simulink model "mavsim_chap4"  (R2018b)
settings: Solver=ode45  StartTime=0.0  StopTime=10000  RelTol=1e-3  EnableMultiTasking=on
PreLoadFcn:
  | param
  | aerosonde
InitFcn:
  | param
  | aerosonde
values from neighbouring files (symbols this model uses):
  q = uu(11)    [drawVehicle.m]    (also in forces_moments.m = x(11))
  r = uu(12)    [drawVehicle.m]    (also in forces_moments.m = x(12))
undefined symbols (not defined in the file or in its folder): drawVehicle, forces_moments, HDBK, Light, MIL, Newton, P, plotmavstatevariables, Raphson, sigbuilder_block
libraries: simulink x4, aerolibwind2 x2, aerolibobsolete x1
settings Model: Creator=beard  LastModifiedBy=xinyizhao
settings DataIOCC: LimitDataPoints=on  SaveFormat=Array  SignalLoggingSaveFormat=ModelDataLogs
settings OptimizationCC: ExpressionDepthLimit=2147483647  InitFltsAndDblsToZero=on  LifeSpan=inf
settings DebuggingCC: UnderspecifiedInitializationDetection=Classic  MergeDetectMultiDrivingBlocksExec=none  SolverPrmCheckMsg=warning  FcnCallInpInsideContextMsg=warning  StateNameClashWarn=warning  LibraryContextMissingDiagnostic=none  SFUnexpectedBacktrackingDiag=warning  SFNoUnconditionalDefaultTransitionDiag=warning  SFExecutionAtInitializationDiag=none
settings HardwareCC: ProdBitPerPointer=32  ProdBitPerSizeT=32  ProdBitPerPtrDiffT=32  ProdLargestAtomicFloat=None  ProdIntDivRoundTo=Undefined  ProdEndianess=Unspecified  ProdWordSize=32  ProdHWDeviceType=32-bit Generic
settings ModelReferenceCC: PropagateSignalLabelsOutOfModel=off
settings SFSimCC: SimUseLocalCustomCode=off
settings RTWCC: RTWUseLocalCustomCode=off
settings CodeAppCC: StateflowObjectComments=on
settings GRTTargetCC: TargetLangStandard=C89/C90 (ANSI)  GeneratePreprocessorConditionals=Disable all  CombineOutputUpdateFcns=off  GRTInterface=on
settings ConfigComp: CovMetricSettings=dw  CovHtmlReporting=on  CovSaveCumulativeToWorkspaceVar=on  CovSaveSingleToWorkspaceVar=on  CovExternalEMLEnable=off  CovSFcnEnable=off

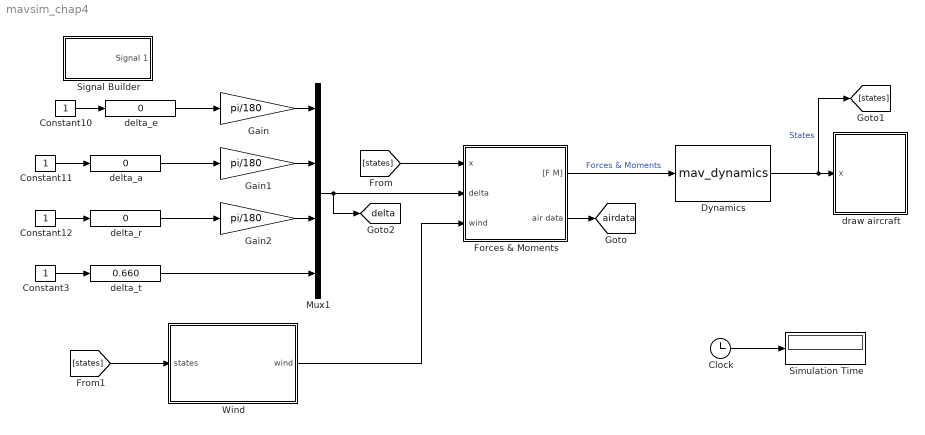
== system mavsim_chap4 ==
  Clock : Clock
  Constant{3,10..12} (4 alike) : Constant
  Dynamics : S-Function  FunctionName=mav_dynamics  Parameters=P  SFunctionDeploymentMode=off  EnableBusSupport=off
  Forces & Moments : Subsystem
  Gain : Gain  Gain=pi/180
  Gain1 : Gain  Gain=pi/180
  Gain2 : Gain  Gain=pi/180
  Mux1 : Mux
  Signal Builder : Subsystem  Tag=STV Subsys  LoadFcn=sigbuilder_block('load');  StartFcn=sigbuilder_block('start');  StopFcn=sigbuilder_block('stop');  ClipboardFcn=sigbuilder_block('clipboard');  mask(Sigbuilder block){tuvar=[0:10]}
      mask help: Simulink:masks:SigbuilderBlock_MD
      mask init:
      | if ~strcmp(get_param(bdroot(gcbh),'SimulationStatus'),'stopped') tuvar = sigbuilder_block('maskInit'); end
      settings: CopyFcn=sigbuilder_block('copy');  DeleteFcn=sigbuilder_block('delete');  ModelCloseFcn=sigbuilder_block('modelClose');  PreSaveFcn=sigbuilder_block('preSave');  PauseFcn=sigbuilder_block('pause');  ContinueFcn=sigbuilder_block('continue');  NameChangeFcn=sigbuilder_block('namechange');  OpenFcn=sigbuilder_block('open',[382.5 81 550.5 358.5 ]);  CloseFcn=sigbuilder_block('close');
      mask Display: plot(0, 0, 100, 100,[2, 2, 32, 32, 2], [68, 8, 8, 68, 68],[32, 2], [38, 38], [32, 19, 2],[53, 60, 44], [32, 17, 17, 2],[16, 16, 31, 31]);txt = getActiveGroup(gcbh);text(2, 100, txt,'verticalAlignment', 'top');
  Simulation Time : Display
  Wind : Subsystem
  delta_a : simulink/Math Operations/Slider Gain  gain=0  low=-45  high=45
  delta_e : simulink/Math Operations/Slider Gain  gain=0  low=-45  high=45
  delta_r : simulink/Math Operations/Slider Gain  gain=0  low=-45  high=45
  delta_t : simulink/Math Operations/Slider Gain  gain=0.660  low=0  high=1
  draw aircraft : Subsystem
      mask Display: image(imread('tv.jpg'))
  tag scope: airdata=global, delta=global
  wires:
  Constant10/1 -> delta_e/1
  Constant11/1 -> delta_a/1
  Constant12/1 -> delta_r/1
  Dynamics/1 -> [states], draw aircraft/1(x)  "States"
  Constant3/1 -> delta_t/1
  delta_t/1 -> Mux1/4
  Mux1/1 -> [delta], Forces & Moments/2(delta)
  Forces & Moments/1("[F M]") -> Dynamics/1  "Forces & Moments"
  Clock/1 -> Simulation Time/1
  Wind/1(wind) -> Forces & Moments/3(wind)
  Forces & Moments/2(air data) -> [airdata]
  Gain/1 -> Mux1/1
  Gain1/1 -> Mux1/2
  Gain2/1 -> Mux1/3
  [states] -> Forces & Moments/1(x)
  [states] -> Wind/1(states)
  delta_e/1 -> Gain/1
  delta_a/1 -> Gain1/1
  delta_r/1 -> Gain2/1

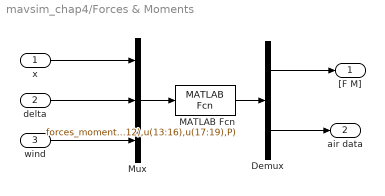
== system mavsim_chap4/Forces & Moments ==
  x : Inport
  delta : Inport  Port=2
  wind : Inport  Port=3
  Demux : Demux  Outputs=[6;6]
  MATLAB Fcn : MATLABFcn  MATLABFcn=forces_moments(u(1:12),u(13:16),u(17:19),P)  OutputDimensions=12
  Mux : Mux  Inputs=3
  "[F M]" : Outport
  air data : Outport  Port=2
  wires:
  x/1 -> Mux/1
  delta/1 -> Mux/2
  wind/1 -> Mux/3
  MATLAB Fcn/1 -> Demux/1
  Demux/1 -> "[F M]"/1
  Mux/1 -> MATLAB Fcn/1
  Demux/2 -> air data/1

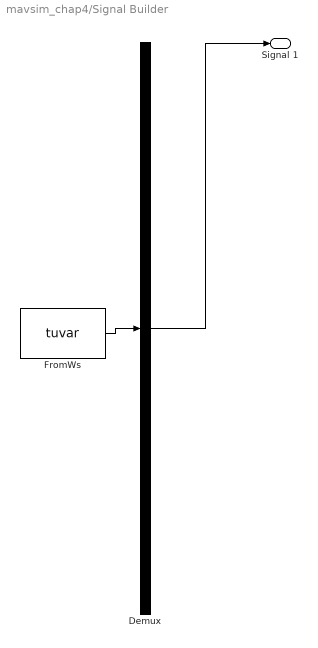
== system mavsim_chap4/Signal Builder ==
  Demux : Demux  Tag=STV Demux  Outputs=1
  FromWs : FromWorkspace  Tag=STV FromWs  VariableName=tuvar  SampleTime=0
      SigBuilderData=|
      | common.afterFinalStr = 'Extrapolate'
      | common.sampleTime = 0
      | dataSet.timeRange = [0 20]
      | dataSet.name = 'Group 1'
      | sbobj.Groups.Name = 'Group 1'
      | sbobj.Groups.Signals.Name = 'Signal 1'
      | sbobj.Groups.Signals.XData = [0 10 10 15 15 20]
      | sbobj.Groups.Signals.YData = [0 0 5 5 0 0]
      | sbobj.Groups.TimeRange = [0 20]
  Signal 1 : Outport  Tag=STV Outport
  wires:
  Demux/1 -> Signal 1/1
  FromWs/1 -> Demux/1

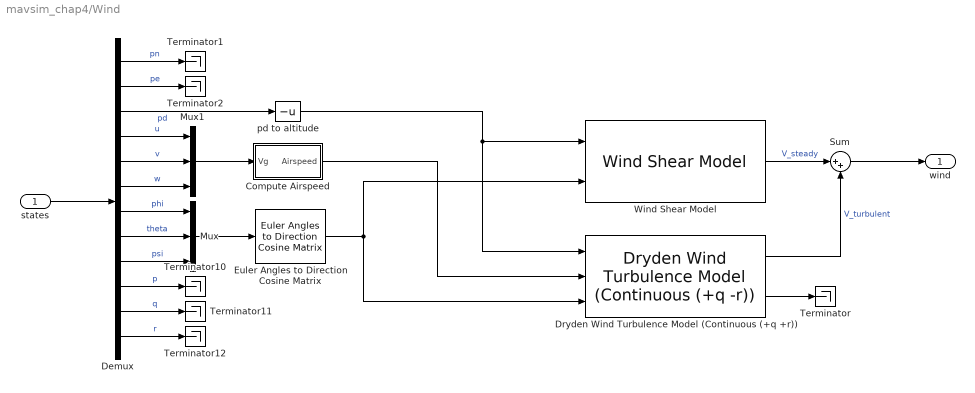
== system mavsim_chap4/Wind ==
  states : Inport
  Compute Airspeed : Subsystem
  Demux : Demux  Outputs=12
  Dryden Wind Turbulence Model (Continuous (+q +r)) : aerolibwind2/Dryden Wind Turbulence Model  (Continuous (+q -r))  units=Metric (MKS)  spec=MIL-HDBK-1797  model=Continuous Dryden (+q +r)  W20=P.w_mag  Wdeg=P.w_dir  TurbProb=10^-2 - Light  L_high=533.4  Wingspan=P.b  ts=0.1  Seed=[23341 23342 0 23344]  T_on=off
      settings: SourceProductName=Aerospace Blockset
  Euler Angles to Direction Cosine Matrix : aerolibobsolete/Euler Angles to  Direction Cosine Matrix
      settings: SourceProductName=Aerospace Blockset  SourceProductBaseCode=AE
  Mux : Mux  Inputs=3
  Mux1 : Mux  Inputs=3
  Sum : Sum  Inputs=|++
  Terminator{,1..2,10..12} (6 alike) : Terminator
  Wind Shear Model : aerolibwind2/Wind Shear Model  units=Metric (MKS)  phase=Category C - Terminal Flight Phase  W_20=P.w_mag  Wdeg=P.w_dir
      settings: SourceProductName=Aerospace Blockset
  pd to altitude : UnaryMinus
  wind : Outport
  wires:
  Dryden Wind Turbulence Model (Continuous (+q +r))/2 -> Terminator/1
  Euler Angles to Direction Cosine Matrix/1 -> Dryden Wind Turbulence Model (Continuous (+q +r))/3, Wind Shear Model/2
  Wind Shear Model/1 -> Sum/1  "V_steady"
  Compute Airspeed/1(Airspeed) -> Dryden Wind Turbulence Model (Continuous (+q +r))/2
  pd to altitude/1 -> Wind Shear Model/1, Dryden Wind Turbulence Model (Continuous (+q +r))/1
  Dryden Wind Turbulence Model (Continuous (+q +r))/1 -> Sum/2  "V_turbulent"
  states/1 -> Demux/1
  Demux/1 -> Terminator1/1  "pn"
  Demux/2 -> Terminator2/1  "pe"
  Demux/3 -> pd to altitude/1  "pd"
  Demux/4 -> Mux1/1  "u"
  Demux/5 -> Mux1/2  "v"
  Demux/6 -> Mux1/3  "w"
  Demux/7 -> Mux/1  "phi"
  Demux/8 -> Mux/2  "theta"
  Demux/9 -> Mux/3  "psi"
  Demux/10 -> Terminator10/1  "p"
  Demux/11 -> Terminator11/1  "q"
  Demux/12 -> Terminator12/1  "r"
  Mux/1 -> Euler Angles to Direction Cosine Matrix/1
  Mux1/1 -> Compute Airspeed/1(Vg)
  Sum/1 -> wind/1

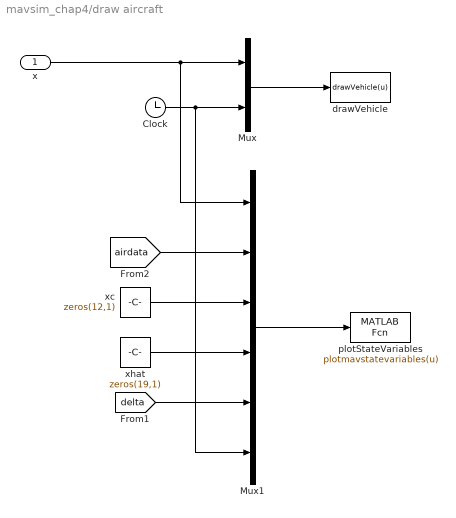
== system mavsim_chap4/draw aircraft ==
  x : Inport
  Clock : Clock
  Mux : Mux  Inputs=2
  Mux1 : Mux  Inputs=6
  drawVehicle : MATLABFcn  MATLABFcn=drawVehicle(u)  OutputDimensions=0  SampleTime=0.1
  plotStateVariables : MATLABFcn  MATLABFcn=plotmavstatevariables(u)  OutputDimensions=0  SampleTime=0.1
  xc : Constant  Value=zeros(12,1)
  xhat : Constant  Value=zeros(19,1)
  wires:
  [airdata] -> Mux1/2
  [delta] -> Mux1/5
  xc/1 -> Mux1/3
  xhat/1 -> Mux1/4
  Mux1/1 -> plotStateVariables/1
  Clock/1 -> Mux1/6, Mux/2
  x/1 -> Mux1/1, Mux/1
  Mux/1 -> drawVehicle/1

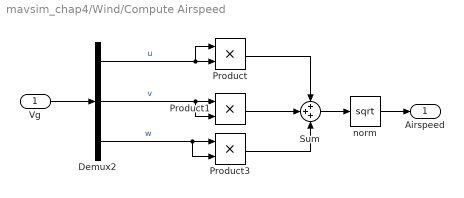
== system mavsim_chap4/Wind/Compute Airspeed ==
  Vg : Inport
  Demux2 : Demux  Outputs=3
  Product : Product  RndMeth=Zero
  Product1 : Product  RndMeth=Zero
  Product3 : Product  RndMeth=Zero
  Sum : Sum  Inputs=+++
  norm : Sqrt  AlgorithmType=Newton-Raphson  SaturateOnIntegerOverflow=on
  Airspeed : Outport
  wires:
  Vg/1 -> Demux2/1
  Product/1 -> Sum/1
  Sum/1 -> norm/1
  Demux2/1 -> Product/2, Product/1  "u"
  Product1/1 -> Sum/2
  Product3/1 -> Sum/3
  Demux2/2 -> Product1/2, Product1/1  "v"
  Demux2/3 -> Product3/2, Product3/1  "w"
  norm/1 -> Airspeed/1
